simulink model "LAB1_1_sim"  (R2025b)
settings: Solver=VariableStepAuto  StartTime=0.0  StopTime=6  RelTol=1e-3
undefined symbols (not defined in the file or in its folder): BEMF_comp, Beq, daq, drv, Fri_comp, gbox, In_comp, Jeq, Kd, Ki, Kp, Kw, mot, om_comp, pulse2deg, rads2rpm, Req, tau_sf_est, Tausf, Tl
libraries: simulink x1
settings Model: Creator=Gioele  LastModifiedBy=super
settings DataIOCC: ReturnWorkspaceOutputs=off

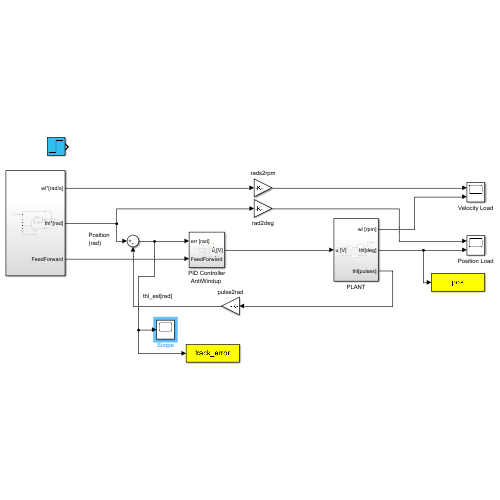
[thumbnail: Simulink's stored preview of the top-level diagram]
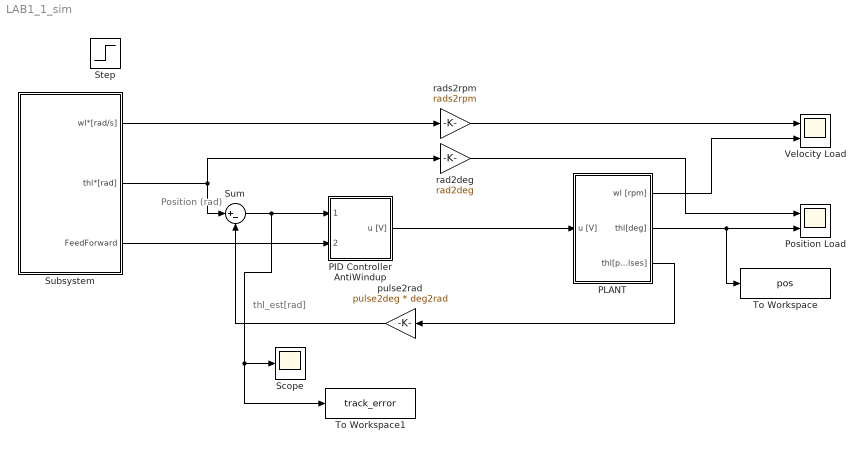
== system LAB1_1_sim ==
  note: thl_est[rad]
  note: Position
      | (rad)
  "PID Controller AntiWindup " : Subsystem
  PLANT : Subsystem
  Position Load : Scope  NumInputPorts=2
      settings: ActiveDisplayYMinimum=-348.38121687666273  ActiveDisplayYMaximum=3049.4145821110656
  Scope : Scope
      settings: ActiveDisplayYMinimum=-0.143270264800738  ActiveDisplayYMaximum=0.14156000805572422  DataLoggingVariableName=ScopeData3
  Step : Step  After=360*(pi/180)  SampleTime=0
  Subsystem : Subsystem
  Sum : Sum  Inputs=|+-
  To Workspace : ToWorkspace  VariableName=pos  SaveFormat=Structure With Time  SampleTime=-1
  To Workspace1 : ToWorkspace  VariableName=track_error  SaveFormat=Structure With Time  SampleTime=-1
  Velocity Load : Scope  NumInputPorts=2
      settings: ActiveDisplayYMinimum=418.8599  ActiveDisplayYMaximum=462.8738
  pulse2rad : Gain  Gain=pulse2deg * deg2rad
  rad2deg : Gain  Gain=rad2deg
  rads2rpm : Gain  Gain=rads2rpm
  wires:
  Sum/1 -> To Workspace1/1, Scope/1, "PID Controller AntiWindup "/1(err [rad])
  Subsystem/2(thl*[rad]) -> Sum/1, rad2deg/1
  pulse2rad/1 -> Sum/2
  rads2rpm/1 -> Velocity Load/1
  Subsystem/1(wl*[rad/s]) -> rads2rpm/1
  Subsystem/3(FeedForward) -> "PID Controller AntiWindup "/2(FeedForward)
  "PID Controller AntiWindup "/1(u [V]) -> PLANT/1(u [V])
  PLANT/1(wl [rpm]) -> Velocity Load/2
  PLANT/2(thl[deg]) -> To Workspace/1, Position Load/2
  PLANT/3(thl[pulses]) -> pulse2rad/1
  rad2deg/1 -> Position Load/1

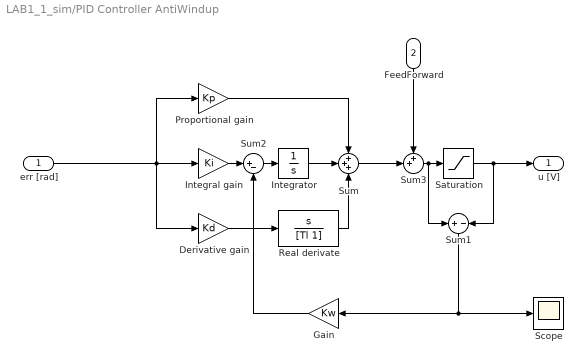
== system LAB1_1_sim/PID Controller AntiWindup  ==
  err [rad] : Inport
  FeedForward : Inport  Port=2
  Derivative gain : Gain  Gain=Kd
  Gain : Gain  Gain=Kw
  "Integral gain " : Gain  Gain=Ki
  Integrator : Integrator
  Proportional gain : Gain  Gain=Kp
  Real derivate : TransferFcn  Numerator=[1 0]  Denominator=[Tl 1]
  Saturation : Saturate  UpperLimit=daq.dac.fs  LowerLimit=-daq.dac.fs
  Scope : Scope
      settings: ActiveDisplayYMinimum=-1  ActiveDisplayYMaximum=1  DataLoggingVariableName=ScopeData2
  Sum : Sum  Inputs=+++
  Sum1 : Sum  Inputs=+|-
  Sum2 : Sum  Inputs=|+-
  Sum3 : Sum  Inputs=++|
  u [V] : Outport
  wires:
  Real derivate/1 -> Sum/3
  Integrator/1 -> Sum/2
  err [rad]/1 -> Proportional gain/1, Derivative gain/1, "Integral gain "/1
  Proportional gain/1 -> Sum/1
  Derivative gain/1 -> Real derivate/1
  Saturation/1 -> Sum1/2, u [V]/1
  Sum1/1 -> Scope/1, Gain/1
  "Integral gain "/1 -> Sum2/1
  Sum2/1 -> Integrator/1
  Gain/1 -> Sum2/2
  Sum3/1 -> Sum1/1, Saturation/1
  Sum/1 -> Sum3/2
  FeedForward/1 -> Sum3/1

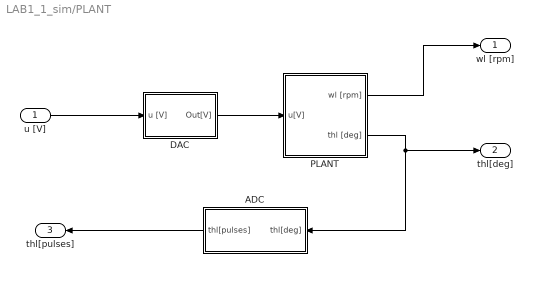
== system LAB1_1_sim/PLANT ==
  u [V] : Inport
  ADC : Subsystem  TreatAsAtomicUnit=on
  DAC : Subsystem  TreatAsAtomicUnit=on
  PLANT : Subsystem
  wl [rpm] : Outport
  thl[deg] : Outport  Port=2
  thl[pulses] : Outport  Port=3
  wires:
  u [V]/1 -> DAC/1(u [V])
  PLANT/1(wl [rpm]) -> wl [rpm]/1
  PLANT/2(thl [deg]) -> ADC/1(thl[deg]), thl[deg]/1
  ADC/1(thl[pulses]) -> thl[pulses]/1
  DAC/1(Out[V]) -> PLANT/1(u[V])

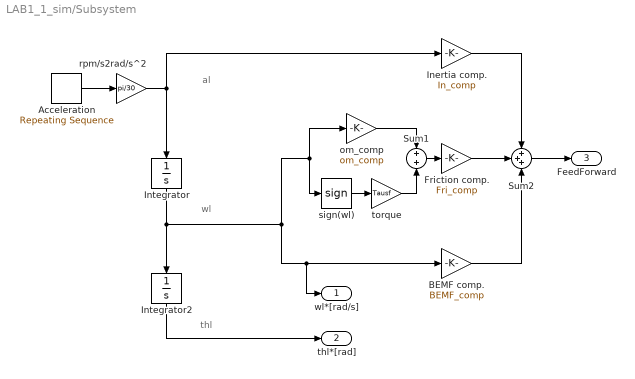
== system LAB1_1_sim/Subsystem ==
  note: al
  note: thl
  note: wl
  Acceleration : simulink/Sources/Repeating Sequence  rep_seq_t=[0, 0.5, 0.50001, 1, 1.0001, 2, 2.0001, 2.5, 2.50001, 3]  rep_seq_y=[900, 900, 0, 0, -900, -900, 0, 0, 900, 900]
  BEMF comp. : Gain  Gain=BEMF_comp
  Friction comp. : Gain  Gain=Fri_comp
  Inertia comp. : Gain  Gain=In_comp
  Integrator : Integrator
  Integrator2 : Integrator
  Sum1 : Sum
  Sum2 : Sum  Inputs=+++
  om_comp : Gain  Gain=om_comp
  rpm/s2rad/s^2 : Gain  Gain=pi/30
  sign(wl) : Signum  ZeroCross=off
  torque : Gain  Gain=Tausf
  wl*[rad/s] : Outport
  thl*[rad] : Outport  Port=2
  FeedForward : Outport  Port=3
  wires:
  sign(wl)/1 -> torque/1
  Acceleration/1 -> rpm/s2rad/s^2/1
  torque/1 -> Sum1/2
  Integrator/1 -> wl*[rad/s]/1, BEMF comp./1, sign(wl)/1, om_comp/1, Integrator2/1
  om_comp/1 -> Sum1/1
  Sum1/1 -> Friction comp./1
  rpm/s2rad/s^2/1 -> Inertia comp./1, Integrator/1
  Inertia comp./1 -> Sum2/1
  Friction comp./1 -> Sum2/2
  BEMF comp./1 -> Sum2/3
  Integrator2/1 -> thl*[rad]/1
  Sum2/1 -> FeedForward/1

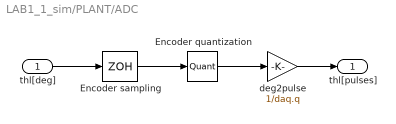
== system LAB1_1_sim/PLANT/ADC ==
  thl[deg] : Inport
  Encoder quantization : Quantizer  QuantizationInterval=daq.q
  Encoder sampling : ZeroOrderHold  SampleTime=daq.dac.Ts
  deg2pulse : Gain  Gain=1/daq.q
  thl[pulses] : Outport
  wires:
  Encoder quantization/1 -> deg2pulse/1
  thl[deg]/1 -> Encoder sampling/1
  Encoder sampling/1 -> Encoder quantization/1
  deg2pulse/1 -> thl[pulses]/1

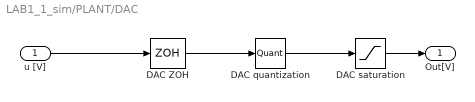
== system LAB1_1_sim/PLANT/DAC ==
  u [V] : Inport
  "DAC ZOH " : ZeroOrderHold  SampleTime=daq.dac.Ts
  DAC quantization : Quantizer  QuantizationInterval=daq.dac.q
  DAC saturation : Saturate  UpperLimit=daq.dac.fs  LowerLimit=-daq.dac.fs
  Out[V] : Outport
  wires:
  DAC quantization/1 -> DAC saturation/1
  u [V]/1 -> "DAC ZOH "/1
  "DAC ZOH "/1 -> DAC quantization/1
  DAC saturation/1 -> Out[V]/1

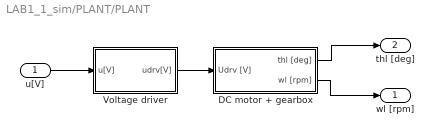
== system LAB1_1_sim/PLANT/PLANT ==
  u[V] : Inport
  DC motor + gearbox : Subsystem
  Voltage driver : Subsystem  TreatAsAtomicUnit=on
  wl [rpm] : Outport
  thl [deg] : Outport  Port=2
  wires:
  Voltage driver/1(udrv[V]) -> DC motor + gearbox/1(Udrv [V])
  u[V]/1 -> Voltage driver/1(u[V])
  DC motor + gearbox/1(thl [deg]) -> thl [deg]/1
  DC motor + gearbox/2(wl [rpm]) -> wl [rpm]/1

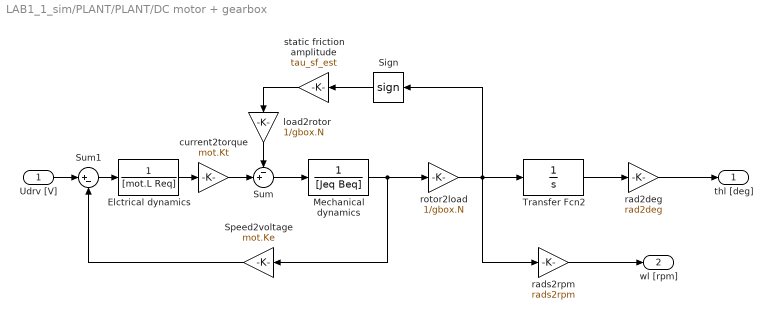
== system LAB1_1_sim/PLANT/PLANT/DC motor + gearbox ==
  Udrv [V] : Inport
  Elctrical dynamics : TransferFcn  Denominator=[mot.L Req]
  Mechanical dynamics : TransferFcn  Denominator=[Jeq Beq]
  Sign : Signum  ZeroCross=off
  Speed2voltage : Gain  Gain=mot.Ke
  Sum : Sum  Inputs=-+|
  Sum1 : Sum  Inputs=|+-
  Transfer Fcn2 : TransferFcn  Denominator=[1 0]
  current2torque : Gain  Gain=mot.Kt
  load2rotor : Gain  Gain=1/gbox.N
  rad2deg : Gain  Gain=rad2deg
  rads2rpm : Gain  Gain=rads2rpm
  rotor2load : Gain  Gain=1/gbox.N
  static friction amplitude : Gain  Gain=tau_sf_est
  thl [deg] : Outport
  wl [rpm] : Outport  Port=2
  wires:
  rotor2load/1 -> Sign/1, rads2rpm/1, Transfer Fcn2/1
  Sign/1 -> static friction amplitude/1
  rads2rpm/1 -> wl [rpm]/1
  Sum/1 -> Mechanical dynamics/1
  Udrv [V]/1 -> Sum1/1
  static friction amplitude/1 -> load2rotor/1
  load2rotor/1 -> Sum/1
  Transfer Fcn2/1 -> rad2deg/1
  current2torque/1 -> Sum/2
  Speed2voltage/1 -> Sum1/2
  Mechanical dynamics/1 -> Speed2voltage/1, rotor2load/1
  Elctrical dynamics/1 -> current2torque/1
  Sum1/1 -> Elctrical dynamics/1
  rad2deg/1 -> thl [deg]/1

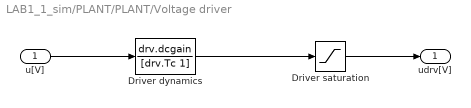
== system LAB1_1_sim/PLANT/PLANT/Voltage driver ==
  u[V] : Inport
  Driver dynamics : TransferFcn  Numerator=drv.dcgain  Denominator=[drv.Tc 1]
  Driver saturation : Saturate  UpperLimit=drv.outmax  LowerLimit=-drv.outmax
  udrv[V] : Outport
  wires:
  Driver dynamics/1 -> Driver saturation/1
  u[V]/1 -> Driver dynamics/1
  Driver saturation/1 -> udrv[V]/1
